simulink model "IndustrialMicrogrid"  (R2023a)
settings: Solver=FixedStepDiscrete  StartTime=0.0  StopTime=10  FixedStep=Ts  RelTol=1e-3
PostLoadFcn:
  | IndustrialMicrogridInputData
  | GfmGridFormingConverterInputParameters
model workspace (MAT data in the model file):
  caseNum = 2
undefined symbols (not defined in the file): base, BESS, DiscIntNeverNeededParam, grid, Grid, gridInverter, machine, microgrid, PV, PVInverter, PVTransformer, scrFactorRg, scrFactorXg, transformer, Ts
libraries: ee_lib x112, eeGeneralControl x104, nesl_utility_internal x64, simulink x56, nesl_utility x37, fl_lib x29, slpidlib x13, eeTransforms x11, eeTotalHarmonicDistorsion x8, eeRmsMeasurement x4, eeSinusoidalMeasurement x4, simulink_extras x2
(part 2 of 14)

== system IndustrialMicrogrid/MG2 PV Plant ==
  (500KWp PV) : Subsystem
      settings: PortSchema="{\"entries\":[{\"content\":{\"sides\":[{\"content\":{\"connectorIds\":[\"Out1\",\"In1\",\"LConn1\"]},\"type\":\"ConnectorPlacement.EquallySpacedRectSide\",\"uuid\":\"7b0e71bf-88d0-4fd9-b424-51733315768d\"},{\"content\":{\"side\":\"RIGHT\"},\"type\":\"ConnectorPlacement.EquallySpacedRectSide\",\"uuid\":\"454a206f-9a61-4ac7-86a8-f6508f61436e\"},{\"content\":{\"side\":\"TOP\"},\"type\":\"ConnectorPlacement.EquallySpacedRectSide\",\"uuid\":\"cf982e1c-b164-4d0a-abcb-f158cc5498a1\"}]},\"type\":\"ConnectorPlacement.EquallySpacedConnector\",\"uuid\":\"7d6089e9-e0b0-4b95-be20-3597ac4fefae\"}],\"packageUris\":[\"http://schema.mathworks.com/mf0/Connector/R2020b\"],\"version\":\"1.0\"}"
  4.16 kV/ 13.8 kV2 : ee_lib/Passive/Transformers/Two-Winding Transformer (Three-Phase)  SRated=PVTransformer.VA A*V  FRated=grid.frequency Hz  Winding1Connection=ee.enum.windingconnection.delta1  VRated1=PVTransformer.hv V  Winding2Connection=ee.enum.windingconnection.Yn  VRated2=PVTransformer.lv V  CoreType=ee.enum.coretype.threelimb  pu_Rw1=PVTransformer.windingResistance*1/2  pu_Rw2=PVTransformer.windingResistance*1/2  leakage_reactance_option=ee.enum.transformer_leakage.include  pu_Xl1=PVTransformer.windingLekageReactance*1/2  pu_Xl2=PVTransformer.windingLekageReactance*1/2  magnetizing_resistance_option=ee.enum.transformer_magnetizingResistance.exclude  pu_Rm=500  magnetizing_reactance_option=ee.enum.transformer_magnetizingReactance.exclude  saturation_option=ee.enum.transformer_saturation.exclude  pu_Xm=500  current_data=[0, .002, 1, 2]  magnetic_flux_data=[0, 1.2, 1.5, 1.51]  pu_X0=PVTransformer.zeroSequenceReactance*1.5  i1_specify=off  i1_priority=None  i1=[0, 0, 0] A  i1_nominal_specify=off  i1_nominal_unit=A  i1_nominal_value=1  i2_specify=off  i2_priority=None  i2=[0, 0, 0] A  i2_nominal_specify=off  i2_nominal_unit=A  i2_nominal_value=1  phi_specify=off  phi_priority=None  phi=[0, 0, 0]  phi_nominal_specify=off  phi_nominal_unit=1  phi_nominal_value=1  power_dissipated_specify=off  power_dissipated_priority=None  power_dissipated=0 W  power_dissipated_nominal_specify=off  power_dissipated_nominal_unit=W  power_dissipated_nominal_value=1
      settings: InternalSimscapePortConfiguration="{\"Bottom\":[],\"Left\":[{\"id\":\"N1\",\"label\":\"~1\",\"type\":\"foundation.electrical.three_phase\"}],\"Right\":[{\"id\":\"N2\",\"label\":\"~2\",\"type\":\"foundation.electrical.three_phase\"},{\"id\":\"n2\",\"label\":\"n2\",\"type\":\"foundation.electrical.electrical\"}],\"Top\":[]}"
  Bus Creator : BusCreator  Inputs=2
  Bus Selector : BusSelector  OutputSignals=Vmag
  CB4 : Subsystem
  Current and Voltage Sensor (Three-Phase)1 : ee_lib/Sensors & Transducers/Current and Voltage Sensor (Three-Phase)  vMeasurementType=ee.enum.vmeasurement.lg  outputUnit=ee.enum.unit.pu  SRated=PV.MVABaseNew A*V  VRated=PV.kVBaseNew V  I_specify=off  I_priority=None  I=[0, 0, 0] A  I_nominal_specify=off  I_nominal_unit=A  I_nominal_value=1  V_specify=off  V_priority=None  V=[0, 0, 0] V  V_nominal_specify=off  V_nominal_unit=V  V_nominal_value=1
      settings: InternalSimscapePortConfiguration="{\"Bottom\":[],\"Left\":[{\"id\":\"N1\",\"label\":\"~1\",\"type\":\"foundation.electrical.three_phase\"}],\"Right\":[{\"id\":\"V_output\",\"label\":\"V\",\"type\":\"output\"},{\"id\":\"I_output\",\"label\":\"I\",\"type\":\"output\"},{\"id\":\"N2\",\"label\":\"~2\",\"type\":\"foundation.electrical.three_phase\"}],\"Top\":[]}"
  Electrical Reference8 : fl_lib/Electrical/Electrical Elements/Electrical Reference
  PLL & Measurements2 : Subsystem
      settings: PortSchema="{\"entries\":[{\"content\":{\"sides\":[{\"content\":{\"connectorIds\":[\"Out1\",\"In1\"]},\"type\":\"ConnectorPlacement.EquallySpacedRectSide\",\"uuid\":\"76485780-20fe-4fcf-8224-69648da6ed2a\"},{\"content\":{\"connectorIds\":[],\"side\":\"RIGHT\"},\"type\":\"ConnectorPlacement.EquallySpacedRectSide\",\"uuid\":\"f19a6390-e634-42c7-8d46-4cd80cbab182\"},{\"content\":{\"connectorIds\":[],\"side\":\"TOP\"},\"type\":\"ConnectorPlacement.EquallySpacedRectSide\",\"uuid\":\"87682f72-1844-428e-be70-ad7ca3191ee3\"}]},\"type\":\"ConnectorPlacement.EquallySpacedConnector\",\"uuid\":\"f2136b07-48ec-402b-adb3-18c0bac2157c\"}],\"packageUris\":[\"http://schema.mathworks.com/mf0/Connector/R2020b\"],\"version\":\"1.0\"}"
  PS-Simulink Converter1 : nesl_utility/PS-Simulink Converter  PhysicalDomain=network_engine_domain  SubClassName=ps_output  LeftPortType=input  RightPortType=output  PseudoPeriodic=off  Frequencies=[]  VectorFormat=inherit  Unit=inherit  AffineConversion=off
  PS-Simulink Converter2 : nesl_utility/PS-Simulink Converter  PhysicalDomain=network_engine_domain  SubClassName=ps_output  LeftPortType=input  RightPortType=output  PseudoPeriodic=off  Frequencies=[]  VectorFormat=inherit  Unit=inherit  AffineConversion=off
  Step : Step  Time=microgrid.controller2PVBrk  Before=1  After=0  SampleTime=Ts
  Terminator : Terminator
  ~ : PMIOPort  Side=Left
  mPV : Outport
  wires:
  (500KWp PV)/1(mPV) -> Bus Creator/1  "mPV"
  PS-Simulink Converter1/1 -> Terminator/1
  Bus Creator/1 -> mPV/1
  Bus Selector/1 -> Bus Creator/2  "<Vmag>"
  Step/1 -> CB4/1(Input)
  PLL & Measurements2/1(Vbus) -> (500KWp PV)/1(Vbus), Bus Selector/1
  PS-Simulink Converter2/1 -> PLL & Measurements2/1(V)
  connections:
  Current and Voltage Sensor (Three-Phase)1/RConn3 -- 4.16 kV/ 13.8 kV2/RConn1
  Current and Voltage Sensor (Three-Phase)1/RConn2 -- PS-Simulink Converter1/LConn1
  CB4/LConn1 -- (500KWp PV)/LConn1
  4.16 kV/ 13.8 kV2/RConn2 -- Electrical Reference8/LConn1
  Current and Voltage Sensor (Three-Phase)1/RConn1 -- PS-Simulink Converter2/LConn1
  Current and Voltage Sensor (Three-Phase)1/LConn1 -- CB4/RConn1
  4.16 kV/ 13.8 kV2/LConn1 -- ~/RConn1

== system IndustrialMicrogrid/MG2 Power Center ==
  Bus Element In3 : Inport  PortName=ControlRoom  Element=PowerCenterBrk1
  Bus Element In1 : Inport  PortName=ControlRoom  Element=PowerCenterBrk2
  Bus Element In2 : Inport  PortName=ControlRoom  Element=PowerCenterDieselBrk
  Bus Element In4 : Inport  PortName=ControlRoom  Element=PowerCenterBrk3
  Circuit Breaker (Three-Phase){,1..3} (4 alike) : ee_lib/Switches & Breakers/Circuit Breaker (Three-Phase)  R_closed=0.001 Ohm  G_open=1e-6 1/Ohm  threshold=0.5 V  breaker_behavior=ee.enum.switches.breakerBehavior.zeroCrossingEnable
      settings: InternalSimscapePortConfiguration="{\"Bottom\":[],\"Left\":[{\"id\":\"vT\",\"label\":\"vT\",\"type\":\"input\"},{\"id\":\"N1\",\"label\":\"~1\",\"type\":\"foundation.electrical.three_phase\"}],\"Right\":[{\"id\":\"N2\",\"label\":\"~2\",\"type\":\"foundation.electrical.three_phase\"}],\"Top\":[]}"
  Diesel Generator : Subsystem
      mask Display: image('$imagefile'); % Use "Edit Image" on toolstrip to change.
  Diesel Measurements : Subsystem
  Fault (Three-Phase) : ee_lib/Utilities/Fault (Three-Phase)  fault_type_option=11  R_pn_fault=1e-3 Ohm  R_ng_fault=1e-3 Ohm  exposemeasurement=ee.enum.exposemeasurement.hidden  enable_external_fault=ee.enum.external_fault.hidden  fault_threshold=0.5  fault_condition=1  fault_resettable=0  enable_temporal_fault=1  fault_start_time=microgrid.controller2PowerCenterFault s  fault_duration=0.1 s  G_parasitic=1e-6 1/Ohm
      settings: InternalSimscapePortConfiguration="{\"Bottom\":[],\"Left\":[{\"id\":\"N\",\"label\":\"~\",\"type\":\"foundation.electrical.three_phase\"}],\"Right\":[],\"Top\":[]}"
  Line X/R=1.44 1 : ee_lib/Passive/RLC Assemblies/RLC (Three-Phase)  component_structure=ee.enum.rlc.structure.SeriesRL  R=microgrid.rLine*0.2 Ohm  L=microgrid.lLine*0.2 H  C=1 F  R_parasitic=1e-6 Ohm  G_parasitic=1e-5 1/Ohm  IL_specify=on  IL_priority=High  IL=[0, 0, 0] A  IL_nominal_specify=off  IL_nominal_unit=A  IL_nominal_value=1  VC_specify=on  VC_priority=High  VC=[0, 0, 0] V  VC_nominal_specify=off  VC_nominal_unit=V  VC_nominal_value=1
      settings: InternalSimscapePortConfiguration="{\"Bottom\":[],\"Left\":[{\"id\":\"N1\",\"label\":\"~1\",\"type\":\"foundation.electrical.three_phase\"}],\"Right\":[{\"id\":\"N2\",\"label\":\"~2\",\"type\":\"foundation.electrical.three_phase\"}],\"Top\":[]}"
  Line X/R=1.44 2 : ee_lib/Passive/RLC Assemblies/RLC (Three-Phase)  component_structure=ee.enum.rlc.structure.SeriesRL  R=microgrid.rLine*0.3 Ohm  L=microgrid.lLine*0.3 H  C=1 F  R_parasitic=1e-6 Ohm  G_parasitic=1e-5 1/Ohm  IL_specify=on  IL_priority=High  IL=[0, 0, 0] A  IL_nominal_specify=off  IL_nominal_unit=A  IL_nominal_value=1  VC_specify=on  VC_priority=High  VC=[0, 0, 0] V  VC_nominal_specify=off  VC_nominal_unit=V  VC_nominal_value=1
      settings: InternalSimscapePortConfiguration="{\"Bottom\":[],\"Left\":[{\"id\":\"N1\",\"label\":\"~1\",\"type\":\"foundation.electrical.three_phase\"}],\"Right\":[{\"id\":\"N2\",\"label\":\"~2\",\"type\":\"foundation.electrical.three_phase\"}],\"Top\":[]}"
  Line X/R=1.44 3 : ee_lib/Passive/RLC Assemblies/RLC (Three-Phase)  component_structure=ee.enum.rlc.structure.SeriesRL  R=microgrid.rLine*0.2 Ohm  L=microgrid.lLine*0.2 H  C=1 F  R_parasitic=1e-6 Ohm  G_parasitic=1e-5 1/Ohm  IL_specify=on  IL_priority=High  IL=[0, 0, 0] A  IL_nominal_specify=off  IL_nominal_unit=A  IL_nominal_value=1  VC_specify=on  VC_priority=High  VC=[0, 0, 0] V  VC_nominal_specify=off  VC_nominal_unit=V  VC_nominal_value=1
      settings: InternalSimscapePortConfiguration="{\"Bottom\":[],\"Left\":[{\"id\":\"N1\",\"label\":\"~1\",\"type\":\"foundation.electrical.three_phase\"}],\"Right\":[{\"id\":\"N2\",\"label\":\"~2\",\"type\":\"foundation.electrical.three_phase\"}],\"Top\":[]}"
  Low-Pass Filter (Discrete or Continuous) : eeGeneralControl/Low-Pass Filter (Discrete or Continuous)  K=1  T=0.1  B=inf  A=-inf  init_option=Inherited from block input  x0=0  Ts=Ts
  Low-Pass Filter (Discrete or Continuous)1 : eeGeneralControl/Low-Pass Filter (Discrete or Continuous)  K=1  T=0.1  B=inf  A=-inf  init_option=Inherited from block input  x0=0  Ts=Ts
  PS-Simulink Converter8 : nesl_utility_internal/PS-Simulink Converter  PhysicalDomain=network_engine_domain  SubClassName=ps_output  LeftPortType=input  RightPortType=output  PseudoPeriodic=off  Frequencies=[]  VectorFormat=1-D array  Unit=MW  AffineConversion=off
  PS-Simulink Converter9 : nesl_utility_internal/PS-Simulink Converter  PhysicalDomain=network_engine_domain  SubClassName=ps_output  LeftPortType=input  RightPortType=output  PseudoPeriodic=off  Frequencies=[]  VectorFormat=1-D array  Unit=MV*A  AffineConversion=off
  Power Sensor (Three-Phase)2 : ee_lib/Sensors & Transducers/Power Sensor (Three-Phase)  load_type=ee.enum.passive.type_balanced.balanced  f0=60 Hz  config=ee.enum.with_neutral.no  rho=1
      settings: InternalSimscapePortConfiguration="{\"Bottom\":[],\"Left\":[{\"id\":\"N1\",\"label\":\"~1\",\"type\":\"foundation.electrical.three_phase\"}],\"Right\":[{\"id\":\"N2\",\"label\":\"~2\",\"type\":\"foundation.electrical.three_phase\"}],\"Top\":[{\"id\":\"Pm\",\"label\":\"P\",\"type\":\"output\"},{\"id\":\"Qm\",\"label\":\"Q\",\"type\":\"output\"}]}"
  Simulink-PS Converter{,1..3} (4 alike) : nesl_utility_internal/Simulink-PS Converter  PhysicalDomain=network_engine_domain  SubClassName=ps_input  LeftPortType=input  RightPortType=output  PseudoPeriodic=off  Frequencies=[]  NoiseDistribution=none  NoiseParameters=[]  Unit=1  AffineConversion=off  FilteringAndDerivatives=provide  SimscapeFilterOrder=1  InputFilterTimeConstant=0.001  UdotUserProvided=0
  Transformer and Disconnectors : Subsystem
      mask Display: image('$imagefile'); % Use "Edit Image" on toolstrip to change.
  Two-Winding Transformer (Three-Phase)1 : ee_lib/Passive/Transformers/Two-Winding Transformer (Three-Phase)  SRated=microgrid.powerCenterTransformerRating A*V  FRated=microgrid.frequency Hz  Winding1Connection=ee.enum.windingconnection.Y  VRated1=microgrid.powerCenterTransformerPrimaryVoltage V  Winding2Connection=ee.enum.windingconnection.Y  VRated2=microgrid.powerCenterTransformerSecondaryVoltage V  CoreType=ee.enum.coretype.threelimb  pu_Rw1=microgrid.powerCenterPrimaryresistance  pu_Rw2=microgrid.powerCenterPrimaryreactance  leakage_reactance_option=ee.enum.transformer_leakage.include  pu_Xl1=microgrid.powerCenterSecondaryresistance  pu_Xl2=microgrid.powerCenterSecondaryreactance  magnetizing_resistance_option=ee.enum.transformer_magnetizingResistance.include  pu_Rm=500  magnetizing_reactance_option=ee.enum.transformer_magnetizingReactance.include  saturation_option=ee.enum.transformer_saturation.exclude  pu_Xm=500  current_data=[0, .002, 1, 2]  magnetic_flux_data=[0, 1.2, 1.5, 1.51]  pu_X0=0.5  i1_specify=on  i1_priority=None  i1=[0, 0, 0] A  i1_nominal_specify=off  i1_nominal_unit=A  i1_nominal_value=1  i2_specify=on  i2_priority=None  i2=[0, 0, 0] A  i2_nominal_specify=off  i2_nominal_unit=A  i2_nominal_value=1  phi_specify=off  phi_priority=None  phi=[0, 0, 0]  phi_nominal_specify=off  phi_nominal_unit=1  phi_nominal_value=1  power_dissipated_specify=off  power_dissipated_priority=None  power_dissipated=0 W  power_dissipated_nominal_specify=off  power_dissipated_nominal_unit=W  power_dissipated_nominal_value=1
      settings: InternalSimscapePortConfiguration="{\"Bottom\":[],\"Left\":[{\"id\":\"N1\",\"label\":\"~1\",\"type\":\"foundation.electrical.three_phase\"}],\"Right\":[{\"id\":\"N2\",\"label\":\"~2\",\"type\":\"foundation.electrical.three_phase\"}],\"Top\":[]}"
  Conn2 : PMIOPort  Side=Left
  ~ a : PMIOPort  Port=2  Side=Left
  " ~ " : PMIOPort  Port=3  Side=Right
  mdiesel : Outport
  Out Bus Element2 : Outport  Port=2  PortName=mtieline  Element=activepower
  Out Bus Element3 : Outport  Port=2  PortName=mtieline  Element=reactivepower
  wires:
  Bus Element In1/1 -> Simulink-PS Converter1/1
  Bus Element In3/1 -> Simulink-PS Converter/1
  Bus Element In2/1 -> Simulink-PS Converter2/1
  Diesel Measurements/1(mdiesel) -> mdiesel/1  "mDiesel"
  Bus Element In4/1 -> Simulink-PS Converter3/1
  PS-Simulink Converter8/1 -> Low-Pass Filter (Discrete or Continuous)/1
  Low-Pass Filter (Discrete or Continuous)1/1 -> Out Bus Element3/1
  PS-Simulink Converter9/1 -> Low-Pass Filter (Discrete or Continuous)1/1
  Low-Pass Filter (Discrete or Continuous)/1 -> Out Bus Element2/1
  connections:
  Line X/R=1.44 1/RConn1 -- Fault (Three-Phase)/LConn1 -- ~ a/RConn1
  Line X/R=1.44 3/RConn1 -- " ~ "/RConn1
  Circuit Breaker (Three-Phase)1/RConn1 -- Two-Winding Transformer (Three-Phase)1/LConn1
  Simulink-PS Converter/RConn1 -- Circuit Breaker (Three-Phase)/LConn1
  Circuit Breaker (Three-Phase)1/LConn2 -- Circuit Breaker (Three-Phase)3/LConn2 -- Circuit Breaker (Three-Phase)/RConn1
  Simulink-PS Converter1/RConn1 -- Circuit Breaker (Three-Phase)1/LConn1
  Line X/R=1.44 2/LConn1 -- Conn2/RConn1
  Diesel Generator/RConn1 -- Transformer and Disconnectors/LConn1
  Simulink-PS Converter2/RConn1 -- Circuit Breaker (Three-Phase)2/LConn1
  Circuit Breaker (Three-Phase)2/RConn1 -- Two-Winding Transformer (Three-Phase)1/RConn1 -- Line X/R=1.44 3/LConn1
  Transformer and Disconnectors/RConn1 -- Diesel Measurements/LConn1
  Diesel Measurements/RConn1 -- Circuit Breaker (Three-Phase)2/LConn2
  Circuit Breaker (Three-Phase)3/RConn1 -- Line X/R=1.44 1/LConn1
  Simulink-PS Converter3/RConn1 -- Circuit Breaker (Three-Phase)3/LConn1
  PS-Simulink Converter9/LConn1 -- Power Sensor (Three-Phase)2/LConn3
  PS-Simulink Converter8/LConn1 -- Power Sensor (Three-Phase)2/LConn2
  Power Sensor (Three-Phase)2/LConn1 -- Line X/R=1.44 2/RConn1
  Power Sensor (Three-Phase)2/RConn1 -- Circuit Breaker (Three-Phase)/LConn2

== system IndustrialMicrogrid/MG2 Primary Substation ==
  ControlRoom : Inport
  BESS and Controller 2 : Subsystem
  Bus Creator : BusCreator  Inputs=2
  Bus Selector : BusSelector  OutputSignals=Substation2Brk
  Circuit Breaker (Three-Phase) : ee_lib/Switches & Breakers/Circuit Breaker (Three-Phase)  R_closed=0.001 Ohm  G_open=1e-6 1/Ohm  threshold=0.5 V  breaker_behavior=ee.enum.switches.breakerBehavior.zeroCrossingEnable
      settings: InternalSimscapePortConfiguration="{\"Bottom\":[],\"Left\":[{\"id\":\"vT\",\"label\":\"vT\",\"type\":\"input\"},{\"id\":\"N1\",\"label\":\"~1\",\"type\":\"foundation.electrical.three_phase\"}],\"Right\":[{\"id\":\"N2\",\"label\":\"~2\",\"type\":\"foundation.electrical.three_phase\"}],\"Top\":[]}"
  Microgrid Controller 2 : Subsystem
  PCC Measurements and PCC Breaker : Subsystem
      mask Display: image('$imagefile'); % Use "Edit Image" on toolstrip to change.
  Simulink-PS Converter : nesl_utility_internal/Simulink-PS Converter  PhysicalDomain=network_engine_domain  SubClassName=ps_input  LeftPortType=input  RightPortType=output  PseudoPeriodic=off  Frequencies=[]  NoiseDistribution=none  NoiseParameters=[]  Unit=1  AffineConversion=off  FilteringAndDerivatives=provide  SimscapeFilterOrder=1  InputFilterTimeConstant=0.001  UdotUserProvided=0
  Transformer and Disconnectors : Subsystem
      mask Display: image('$imagefile'); % Use "Edit Image" on toolstrip to change.
  ~ : PMIOPort  Side=Left
  "~ " : PMIOPort  Port=2  Side=Right
  MGController2 : Outport
  wires:
  Bus Creator/1 -> MGController2/1
  BESS and Controller 2/1(mBESS) -> Bus Creator/1, [BESS2]  "BESS2"
  PCC Measurements and PCC Breaker/1(" mPCC2") -> Microgrid Controller 2/3("mPCC2 ")
  [CtrlRoom] -> Bus Selector/1
  Bus Selector/1 -> Simulink-PS Converter/1  "<Substation2Brk>"
  [CtrlRoom] -> BESS and Controller 2/1(CntrlRmIN)
  [BESS2] -> Microgrid Controller 2/2(BESS 2)
  Microgrid Controller 2/4(MGCtrl) -> [Controller]
  [Controller] -> Bus Creator/2
  ControlRoom/1 -> [CtrlRoom]
  [CtrlRoom] -> Microgrid Controller 2/1(CntrlRmIN)
  Microgrid Controller 2/5(BrkCtrl) -> [cBreaker]
  [cBreaker] -> PCC Measurements and PCC Breaker/1(cBreaker)
  Microgrid Controller 2/1(PQref) -> BESS and Controller 2/2(PQref)
  Microgrid Controller 2/2(Vref) -> BESS and Controller 2/3(Vref)
  Microgrid Controller 2/3(fref) -> BESS and Controller 2/4(f0)
  connections:
  ~/RConn1 -- Transformer and Disconnectors/LConn1
  Transformer and Disconnectors/RConn1 -- PCC Measurements and PCC Breaker/LConn1
  PCC Measurements and PCC Breaker/RConn1 -- Circuit Breaker (Three-Phase)/LConn2 -- BESS and Controller 2/LConn1
  Simulink-PS Converter/RConn1 -- Circuit Breaker (Three-Phase)/LConn1
  "~ "/RConn1 -- Circuit Breaker (Three-Phase)/RConn1

== system IndustrialMicrogrid/MG2 Processing, Lighting and Auxiliary Loads ==
  Bus Element In1 : Inport  PortName=ControlRoom  Element=Load3Control
  Bus Element In4 : Inport  PortName=ControlRoom  Element=Load5Control
  Bus Element In3 : Inport  PortName=ControlRoom  Element=Load4aControl
  Bus Element In2 : Inport  PortName=ControlRoom  Element=Load4bControl
  Circuit Breaker (Three-Phase){1..4} (4 alike) : ee_lib/Switches & Breakers/Circuit Breaker (Three-Phase)  R_closed=0.001 Ohm  G_open=1e-6 1/Ohm  threshold=0.5 V  breaker_behavior=ee.enum.switches.breakerBehavior.zeroCrossingEnable
      settings: InternalSimscapePortConfiguration="{\"Bottom\":[],\"Left\":[{\"id\":\"vT\",\"label\":\"vT\",\"type\":\"input\"},{\"id\":\"N1\",\"label\":\"~1\",\"type\":\"foundation.electrical.three_phase\"}],\"Right\":[{\"id\":\"N2\",\"label\":\"~2\",\"type\":\"foundation.electrical.three_phase\"}],\"Top\":[]}"
  Electrical Reference1 : fl_lib/Electrical/Electrical Elements/Electrical Reference
  Electrical Reference2 : fl_lib/Electrical/Electrical Elements/Electrical Reference
  Electrical Reference5 : fl_lib/Electrical/Electrical Elements/Electrical Reference
  Load Measurements1 : Subsystem
      settings: PortSchema="{\"entries\":[{\"content\":{\"sides\":[{\"content\":{\"connectorIds\":[\"LConn1\"]},\"type\":\"ConnectorPlacement.EquallySpacedRectSide\",\"uuid\":\"d870a913-f96e-493f-ac0f-f00d694ce040\"},{\"content\":{\"connectorIds\":[\"Out1\"],\"side\":\"RIGHT\"},\"type\":\"ConnectorPlacement.EquallySpacedRectSide\",\"uuid\":\"12eea89c-1ef8-4155-8c58-3c970c5d9b18\"},{\"content\":{\"connectorIds\":[],\"side\":\"TOP\"},\"type\":\"ConnectorPlacement.EquallySpacedRectSide\",\"uuid\":\"8c8b4bd0-9ee8-4a98-bcb2-09acde5bae56\"},{\"content\":{\"connectorIds\":[\"RConn1\"],\"side\":\"BOTTOM\"},\"type\":\"ConnectorPlacement.EquallySpacedRectSide\",\"uuid\":\"443bcb6e-ffa1-4f95-8c19-122149ac17cf\"}]},\"type\":\"ConnectorPlacement.EquallySpacedConnector\",\"uuid\":\"4cf8469f-5e58-4383-9537-851b6a4abf90\"}],\"packageUris\":[\"http://schema.mathworks.com/mf0/Connector/R2020b\"],\"version\":\"1.0\"}"
  Load for auxiliary : ee_lib/Passive/RLC Assemblies/Wye-Connected Load  parameterization=ee.enum.rlc.parameterization.ratedpower  component_structure=ee.enum.rlc.structure.C  component_structure_PQ=ee.enum.rlc.structure.SeriesRL  R=1 Ohm  L=0.001 H  C=1e-6 F  VRated=microgrid.powerCenterVoltage V  FRated=microgrid.frequency Hz  P=microgrid.pLoad22 W  Qpos=microgrid.qLoad22 A*V  Qneg=-3000 A*V  R_parasitic=1e-6 Ohm  G_parasitic=1e-6 1/Ohm  R_parasitic_PQ=1e-6 Ohm  G_parasitic_PQ=1e-6 1/Ohm  Vmag0=0 V  Vang0=0 deg  Freq0=microgrid.frequency Hz  IL_specify=on  IL_priority=High  IL=[ 0 0 0 ] A  IL_nominal_specify=off  IL_nominal_unit=A  IL_nominal_value=1  VC_specify=on  VC_priority=High  VC=[ 0 0 0 ] V  VC_nominal_specify=off  VC_nominal_unit=V  VC_nominal_value=1
  Load for auxiliary1 : ee_lib/Passive/RLC Assemblies/Wye-Connected Load  parameterization=ee.enum.rlc.parameterization.ratedpower  component_structure=ee.enum.rlc.structure.C  component_structure_PQ=ee.enum.rlc.structure.SeriesRL  R=1 Ohm  L=0.001 H  C=1e-6 F  VRated=microgrid.powerCenterVoltage V  FRated=microgrid.frequency Hz  P=microgrid.pLoad33 W  Qpos=microgrid.qLoad33 A*V  Qneg=-3000 A*V  R_parasitic=1e-6 Ohm  G_parasitic=1e-6 1/Ohm  R_parasitic_PQ=1e-6 Ohm  G_parasitic_PQ=1e-6 1/Ohm  Vmag0=0 V  Vang0=0 deg  Freq0=microgrid.frequency Hz  IL_specify=on  IL_priority=High  IL=[ 0 0 0 ] A  IL_nominal_specify=off  IL_nominal_unit=A  IL_nominal_value=1  VC_specify=on  VC_priority=High  VC=[ 0 0 0 ] V  VC_nominal_specify=off  VC_nominal_unit=V  VC_nominal_value=1
  Load for lights : ee_lib/Passive/RLC Assemblies/Wye-Connected Load  parameterization=ee.enum.rlc.parameterization.ratedpower  component_structure=ee.enum.rlc.structure.C  component_structure_PQ=ee.enum.rlc.structure.SeriesRL  R=1 Ohm  L=0.001 H  C=1e-6 F  VRated=microgrid.powerCenterVoltage V  FRated=microgrid.frequency Hz  P=microgrid.pLoad21 W  Qpos=microgrid.qLoad21 A*V  Qneg=-3000 A*V  R_parasitic=1e-6 Ohm  G_parasitic=1e-6 1/Ohm  R_parasitic_PQ=1e-6 Ohm  G_parasitic_PQ=1e-6 1/Ohm  Vmag0=0 V  Vang0=0 deg  Freq0=microgrid.frequency Hz  IL_specify=on  IL_priority=High  IL=[ 0 0 0 ] A  IL_nominal_specify=off  IL_nominal_unit=A  IL_nominal_value=1  VC_specify=on  VC_priority=High  VC=[ 0 0 0 ] V  VC_nominal_specify=off  VC_nominal_unit=V  VC_nominal_value=1
  Motor Loads : Subsystem
  RLC (Three-Phase) : ee_lib/Passive/RLC Assemblies/RLC (Three-Phase)  component_structure=ee.enum.rlc.structure.SeriesRL  R=1 Ohm  L=5e-3 H  C=1e-6 F  R_parasitic=0 Ohm  G_parasitic=0 1/Ohm  IL_specify=off  IL_priority=High  IL=[0, 0, 0] A  IL_nominal_specify=off  IL_nominal_unit=A  IL_nominal_value=1  VC_specify=off  VC_priority=High  VC=[0, 0, 0] V  VC_nominal_specify=off  VC_nominal_unit=V  VC_nominal_value=1
      settings: InternalSimscapePortConfiguration="{\"Bottom\":[],\"Left\":[{\"id\":\"N1\",\"label\":\"~1\",\"type\":\"foundation.electrical.three_phase\"}],\"Right\":[{\"id\":\"N2\",\"label\":\"~2\",\"type\":\"foundation.electrical.three_phase\"}],\"Top\":[]}"
  Simulink-PS Converter{1..4} (4 alike) : nesl_utility_internal/Simulink-PS Converter  PhysicalDomain=network_engine_domain  SubClassName=ps_input  LeftPortType=input  RightPortType=output  PseudoPeriodic=off  Frequencies=[]  NoiseDistribution=none  NoiseParameters=[]  Unit=1  AffineConversion=off  FilteringAndDerivatives=provide  SimscapeFilterOrder=1  InputFilterTimeConstant=0.001  UdotUserProvided=0
  ~ : PMIOPort  Side=Left
  mLoad2 : Outport
  wires:
  Load Measurements1/1(mLoad2) -> mLoad2/1
  Bus Element In1/1 -> Simulink-PS Converter3/1
  Bus Element In3/1 -> Simulink-PS Converter1/1
  Bus Element In4/1 -> Simulink-PS Converter2/1
  Bus Element In2/1 -> Simulink-PS Converter4/1
  connections:
  Electrical Reference2/LConn1 -- Load for lights/RConn1
  Simulink-PS Converter3/RConn1 -- Circuit Breaker (Three-Phase)1/LConn1
  Simulink-PS Converter1/RConn1 -- Circuit Breaker (Three-Phase)2/LConn1
  ~/RConn1 -- Load Measurements1/LConn1
  Circuit Breaker (Three-Phase)1/RConn1 -- Load for lights/LConn1
  Load for auxiliary/LConn1 -- Circuit Breaker (Three-Phase)2/RConn1
  Load for auxiliary/RConn1 -- Electrical Reference5/LConn1
  RLC (Three-Phase)/RConn1 -- Circuit Breaker (Three-Phase)3/LConn2
  Simulink-PS Converter2/RConn1 -- Circuit Breaker (Three-Phase)3/LConn1
  Load Measurements1/RConn1 -- Circuit Breaker (Three-Phase)2/LConn2 -- Circuit Breaker (Three-Phase)4/LConn2 -- RLC (Three-Phase)/LConn1 -- Circuit Breaker (Three-Phase)1/LConn2
  Load for auxiliary1/RConn1 -- Electrical Reference1/LConn1
  Load for auxiliary1/LConn1 -- Circuit Breaker (Three-Phase)4/RConn1
  Simulink-PS Converter4/RConn1 -- Circuit Breaker (Three-Phase)4/LConn1
  Motor Loads/RConn1 -- Circuit Breaker (Three-Phase)3/RConn1

== system IndustrialMicrogrid/Operator Room ==
  mLoad : Inport
  MGController1 : Inport  Port=2
  mTieline1 : Inport  Port=3
  MGController2 : Inport  Port=4
  mPV : Inport  Port=5
  mPowerCenter : Inport  Port=6
  mLoad2 : Inport  Port=7
  mLoad3 : Inport  Port=8
  Bus Creator : BusCreator  Inputs=9
  Bus Creator1 : BusCreator  Inputs=7
  Bus Selector7 : BusSelector  OutputSignals=mDiesel,mTieline
  OperatorControlRoom : Subsystem
      settings: PortSchema="{\"entries\":[{\"content\":{\"sides\":[{\"content\":{\"connectorIds\":[\"Out1\",\"Out2\"]},\"type\":\"ConnectorPlacement.EquallySpacedRectSide\",\"uuid\":\"36e3c748-e70d-4376-8c54-bee35c2cf55e\"},{\"content\":{\"connectorIds\":[\"In1\",\"In2\",\"In3\",\"In4\",\"In5\",\"In6\",\"In7\",\"In8\",\"In9\"],\"side\":\"RIGHT\"},\"type\":\"ConnectorPlacement.EquallySpacedRectSide\",\"uuid\":\"3af4b9ea-3351-4c6c-90c1-760bf6d2a862\"},{\"content\":{\"side\":\"TOP\"},\"type\":\"ConnectorPlacement.EquallySpacedRectSide\",\"uuid\":\"c84439f5-3dbb-4f33-afb8-95498296d6fa\"}]},\"type\":\"ConnectorPlacement.EquallySpacedConnector\",\"uuid\":\"cafa6b3a-2446-4c45-9268-4fc6f6c2350c\"}],\"packageUris\":[\"http://schema.mathworks.com/mf0/Connector/R2020b\"],\"version\":\"1.0\"}"
  Signal Selector : Subsystem
  OperatorRoom : Outport
  OperatorRoomResult : Outport  Port=2
  wires:
  Signal Selector/6("Processing, and Auxiliary Loads ") -> Bus Creator1/6  "Auxiliary Loads"
  MGController2/1 -> Bus Creator/3, OperatorControlRoom/3(MGController2)  "MGController2"
  OperatorControlRoom/1(Control Room MG1) -> Signal Selector/1(Control Room MG1)
  Signal Selector/5(Drilling Load) -> Bus Creator1/5  "Drilling Load"
  Signal Selector/4(Power Center) -> Bus Creator1/4  "Power Center"
  Bus Selector7/1 -> Bus Creator/8, OperatorControlRoom/8(mDiesel)  "<mDiesel>"
  Signal Selector/1(Primary Substation 1) -> Bus Creator1/1  "Primary Substation 1"
  MGController1/1 -> Bus Creator/5, OperatorControlRoom/5(MGController1)  "MGController1"
  mLoad2/1 -> Bus Creator/2, OperatorControlRoom/2(mLoad2)  "mLoad2"
  mLoad/1 -> Bus Creator/1, OperatorControlRoom/1(mLoad)  "mLoad"
  mPV/1 -> Bus Creator/4, OperatorControlRoom/4(mPV)  "mPV"
  Signal Selector/3(Unit Substation) -> Bus Creator1/3  "Unit Substation"
  Signal Selector/7(Portable Substation) -> Bus Creator1/7  "Portable Substation"
  Signal Selector/2(Primary Substation 2) -> Bus Creator1/2  "Primary Substation 2"
  OperatorControlRoom/2(Control Room MG2) -> Signal Selector/2(Control Room MG2)
  mLoad3/1 -> Bus Creator/7, OperatorControlRoom/7(mLoad3)  "mLoad3"
  mPowerCenter/1 -> Bus Selector7/1  "PowerCenter"
  Bus Selector7/2 -> Bus Creator/9, OperatorControlRoom/9(Tieline)  "<mTieline>"
  Bus Creator1/1 -> OperatorRoom/1
  mTieline1/1 -> Bus Creator/6, OperatorControlRoom/6(Tieline1)  "mTieline1"
  Bus Creator/1 -> OperatorRoomResult/1

== system IndustrialMicrogrid/Selected Results ==
  OperatorRoom : Inport
  Bus Selector1 : BusSelector  OutputSignals=MGController2,mLoad2,mPV,mDiesel
  Bus Selector7 : BusSelector  OutputSignals=MGController1,mLoad
  MG1 : Subsystem
  MG2 : Subsystem
  OperatorRoom1 : InportShadow
  wires:
  Bus Selector7/2 -> MG1/2(mLoad)  "<mLoad>"
  Bus Selector7/1 -> MG1/1(MGController1)  "<MGController1>"
  Bus Selector1/1 -> MG2/1(MGController2)  "<MGController2>"
  Bus Selector1/2 -> MG2/2(mLoad2)  "<mLoad2>"
  Bus Selector1/3 -> MG2/3(mPV)  "<mPV>"
  Bus Selector1/4 -> MG2/4(mdiesel)  "<mDiesel>"
  OperatorRoom/1 -> Bus Selector7/1
  OperatorRoom1/1 -> Bus Selector1/1

== system IndustrialMicrogrid/MG1 Drilling Loads/Load Measurements1 ==
  Current and Voltage Sensor (Three-Phase)2 : ee_lib/Sensors & Transducers/Current and Voltage Sensor (Three-Phase)  vMeasurementType=ee.enum.vmeasurement.ll  outputUnit=ee.enum.unit.pu  SRated=1e6 A*V  VRated=microgrid.unitSubstationVoltage V  I_specify=off  I_priority=None  I=[0, 0, 0] A  I_nominal_specify=off  I_nominal_unit=A  I_nominal_value=1  V_specify=off  V_priority=None  V=[0, 0, 0] V  V_nominal_specify=off  V_nominal_unit=V  V_nominal_value=1
      settings: InternalSimscapePortConfiguration="{\"Bottom\":[],\"Left\":[{\"id\":\"N1\",\"label\":\"~1\",\"type\":\"foundation.electrical.three_phase\"}],\"Right\":[{\"id\":\"V_output\",\"label\":\"V\",\"type\":\"output\"},{\"id\":\"I_output\",\"label\":\"I\",\"type\":\"output\"},{\"id\":\"N2\",\"label\":\"~2\",\"type\":\"foundation.electrical.three_phase\"}],\"Top\":[]}"
  Gain : Gain  Gain=sqrt(2)
  Gain1 : Gain  Gain=sqrt(2)
  Line Voltage Sensor (Three-Phase) : ee_lib/Sensors & Transducers/Line Voltage Sensor (Three-Phase)
  Low-Pass Filter (Discrete or Continuous)1 : eeGeneralControl/Low-Pass Filter (Discrete or Continuous)  K=1  T=0.02  B=inf  A=-inf  init_option=Inherited from block input  x0=0  Ts=Ts
  Low-Pass Filter (Discrete or Continuous)2 : eeGeneralControl/Low-Pass Filter (Discrete or Continuous)  K=1  T=0.02  B=inf  A=-inf  init_option=Inherited from block input  x0=0  Ts=Ts
  PS-Simulink Converter : nesl_utility/PS-Simulink Converter  PhysicalDomain=network_engine_domain  SubClassName=ps_output  LeftPortType=input  RightPortType=output  PseudoPeriodic=off  Frequencies=[]  VectorFormat=inherit  Unit=inherit  AffineConversion=off
  PS-Simulink Converter1 : nesl_utility_internal/PS-Simulink Converter  PhysicalDomain=network_engine_domain  SubClassName=ps_output  LeftPortType=input  RightPortType=output  PseudoPeriodic=off  Frequencies=[]  VectorFormat=1-D array  Unit=inherit  AffineConversion=off
  PS-Simulink Converter12 : nesl_utility_internal/PS-Simulink Converter  PhysicalDomain=network_engine_domain  SubClassName=ps_output  LeftPortType=input  RightPortType=output  PseudoPeriodic=off  Frequencies=[]  VectorFormat=1-D array  Unit=V  AffineConversion=off
  PS-Simulink Converter13 : nesl_utility_internal/PS-Simulink Converter  PhysicalDomain=network_engine_domain  SubClassName=ps_output  LeftPortType=input  RightPortType=output  PseudoPeriodic=off  Frequencies=[]  VectorFormat=1-D array  Unit=A  AffineConversion=off
  PS-Simulink Converter2 : nesl_utility_internal/PS-Simulink Converter  PhysicalDomain=network_engine_domain  SubClassName=ps_output  LeftPortType=input  RightPortType=output  PseudoPeriodic=off  Frequencies=[]  VectorFormat=1-D array  Unit=inherit  AffineConversion=off
  PS-Simulink Converter6 : nesl_utility_internal/PS-Simulink Converter  PhysicalDomain=network_engine_domain  SubClassName=ps_output  LeftPortType=input  RightPortType=output  PseudoPeriodic=off  Frequencies=[]  VectorFormat=1-D array  Unit=MW  AffineConversion=off
  PS-Simulink Converter7 : nesl_utility_internal/PS-Simulink Converter  PhysicalDomain=network_engine_domain  SubClassName=ps_output  LeftPortType=input  RightPortType=output  PseudoPeriodic=off  Frequencies=[]  VectorFormat=1-D array  Unit=MV*A  AffineConversion=off
  Power Sensor (Three-Phase)1 : ee_lib/Sensors & Transducers/Power Sensor (Three-Phase)  load_type=ee.enum.passive.type_balanced.balanced  f0=60 Hz  config=ee.enum.with_neutral.no  rho=1
      settings: InternalSimscapePortConfiguration="{\"Bottom\":[],\"Left\":[{\"id\":\"N1\",\"label\":\"~1\",\"type\":\"foundation.electrical.three_phase\"}],\"Right\":[{\"id\":\"N2\",\"label\":\"~2\",\"type\":\"foundation.electrical.three_phase\"}],\"Top\":[{\"id\":\"Pm\",\"label\":\"P\",\"type\":\"output\"},{\"id\":\"Qm\",\"label\":\"Q\",\"type\":\"output\"}]}"
  RMS Measurement : eeRmsMeasurement/RMS Measurement  LabelModeActiveChoice=Total  F=60  SpecifyHarmonics=off  K=[0 1 2]  Ts=Ts
      settings: LibrarySourceBlock=|
      | ee_sl_lib/Measurements/RMS
      | Measurement
  RMS Measurement1 : eeRmsMeasurement/RMS Measurement  LabelModeActiveChoice=Total  F=60  SpecifyHarmonics=off  K=[0 1 2]  Ts=Ts
      settings: LibrarySourceBlock=|
      | ee_sl_lib/Measurements/RMS
      | Measurement
  Scope : Scope
  a2 : PMIOPort  Side=Left
  Conn2 : PMIOPort  Port=2  Side=Right
  Out Bus Element : Outport  PortName=mLoad  Element=active power
  Out Bus Element1 : Outport  PortName=mLoad  Element=reactive power
  Out Bus Element2 : Outport  PortName=mLoad  Element=voltage
  Out Bus Element3 : Outport  PortName=mLoad  Element=current
  Out Bus Element4 : Outport  PortName=mLoad  Element=voltageRMS
  Out Bus Element5 : Outport  PortName=mLoad  Element=currentRMS
  wires:
  PS-Simulink Converter12/1 -> Out Bus Element2/1
  PS-Simulink Converter13/1 -> Out Bus Element3/1
  PS-Simulink Converter7/1 -> Low-Pass Filter (Discrete or Continuous)2/1
  PS-Simulink Converter6/1 -> Low-Pass Filter (Discrete or Continuous)1/1
  PS-Simulink Converter1/1 -> RMS Measurement/1
  PS-Simulink Converter2/1 -> RMS Measurement1/1
  Low-Pass Filter (Discrete or Continuous)1/1 -> Out Bus Element/1
  Low-Pass Filter (Discrete or Continuous)2/1 -> Out Bus Element1/1
  RMS Measurement/1 -> Gain/1
  RMS Measurement1/1 -> Gain1/1
  PS-Simulink Converter/1 -> Scope/1
  Gain/1 -> Out Bus Element4/1
  Gain1/1 -> Out Bus Element5/1
  connections:
  Power Sensor (Three-Phase)1/LConn3 -- PS-Simulink Converter7/LConn1
  Power Sensor (Three-Phase)1/LConn2 -- PS-Simulink Converter6/LConn1
  Current and Voltage Sensor (Three-Phase)2/RConn3 -- Conn2/RConn1
  a2/RConn1 -- Power Sensor (Three-Phase)1/LConn1 -- Line Voltage Sensor (Three-Phase)/LConn1
  Current and Voltage Sensor (Three-Phase)2/RConn1 -- PS-Simulink Converter12/LConn1 -- PS-Simulink Converter1/LConn1
  Current and Voltage Sensor (Three-Phase)2/RConn2 -- PS-Simulink Converter2/LConn1 -- PS-Simulink Converter13/LConn1
  Power Sensor (Three-Phase)1/RConn1 -- Current and Voltage Sensor (Three-Phase)2/LConn1
  PS-Simulink Converter/LConn1 -- Line Voltage Sensor (Three-Phase)/RConn1

== system IndustrialMicrogrid/MG1 Drilling Loads/Subsystem2 ==
  ASM measurement : ee_lib/Electromechanical/Asynchronous/Induction Machine Measurement  output_idx=11
      settings: InternalSimscapePortConfiguration="{\"Bottom\":[],\"Left\":[{\"id\":\"pu_input\",\"label\":\"pu\",\"type\":\"input\"}],\"Right\":[{\"id\":\"pu_output\",\"label\":\"o\",\"type\":\"output\"}],\"Top\":[]}"
  ASM measurement1 : ee_lib/Electromechanical/Asynchronous/Induction Machine Measurement  output_idx=12
      settings: InternalSimscapePortConfiguration="{\"Bottom\":[],\"Left\":[{\"id\":\"pu_input\",\"label\":\"pu\",\"type\":\"input\"}],\"Right\":[{\"id\":\"pu_output\",\"label\":\"o\",\"type\":\"output\"}],\"Top\":[]}"
  ASM measurement2 : ee_lib/Electromechanical/Asynchronous/Induction Machine Measurement  output_idx=12
      settings: InternalSimscapePortConfiguration="{\"Bottom\":[],\"Left\":[{\"id\":\"pu_input\",\"label\":\"pu\",\"type\":\"input\"}],\"Right\":[{\"id\":\"pu_output\",\"label\":\"o\",\"type\":\"output\"}],\"Top\":[]}"
  Asynchronous Machine Squirrel Cage (fundamental) : ee_lib/Electromechanical/Asynchronous/Induction Machine Squirrel Cage  port_option=ee.enum.threePhasePort.composite  SRated=132000 V*A  VRated=microgrid.unitSubstationVoltage V  FRated=grid.frequency Hz  nPolePairs=2  param_unit=ee.enum.unit.si  squirrel_cage=ee.enum.squirrelcage.Single  zero_sequence=ee.enum.park.zerosequence.exclude  initialization_option=ee.enum.asm.initialization.fluxvariables  Rs=0.016744 Ohm  Xls=0.035490 Ohm  pu_Rs=0.0258  pu_Lls=0.0413  Rrd=0.009857 Ohm  Xlrd=0.04280 Ohm  pu_Rrd=0.0145  pu_Llrd=0.0424  Rrd1=0.28 Ohm  Xlrd1=0.82 Ohm  Rrd2=0.28 Ohm  Xlrd2=0.82 Ohm  pu_Rrd1=0.0290  pu_Llrd1=0.0848  pu_Rrd2=0.0290  pu_Llrd2=0.0848  Xm=111.90 Ohm  pu_Lm=1.7562  X0=0.4 Ohm  pu_L0=0.0413  saturation_option=ee.enum.saturation.exclude  saturation_i=[0, 4, 9, 18, 25, 34, 50, 68, 95, 120] A  saturation_v=[0, 88, 154, 198, 220, 242, 264, 286, 308, 327] V  pu_saturation_i=[0, .176, .396, .792, 1.1, 1.496, 2.2, 2.992, 4.18, 5.28]  pu_saturation_v=[0, .4, .7, .9, 1, 1.1, 1.2, 1.3, 1.4, 1.4864]  connection_option=ee.enum.Connection.delta1  angular_position_specify=off  angular_position_priority=None  angular_position=0 deg  angular_position_nominal_specify=off  angular_position_nominal_unit=deg  angular_position_nominal_value=1  pu_psids_specify=off  pu_psids_priority=None  pu_psids=0  pu_psids_nominal_specify=off  pu_psids_nominal_unit=1  pu_psids_nominal_value=1  pu_psiqs_specify=off  pu_psiqs_priority=None  pu_psiqs=0  pu_psiqs_nominal_specify=off  pu_psiqs_nominal_unit=1  pu_psiqs_nominal_value=1  pu_psi0s_specify=off  pu_psi0s_priority=None  pu_psi0s=0  pu_psi0s_nominal_specify=off  pu_psi0s_nominal_unit=1  pu_psi0s_nominal_value=1  pu_psidr_specify=off  pu_psidr_priority=None  pu_psidr=0  pu_psidr_nominal_specify=off  pu_psidr_nominal_unit=1  pu_psidr_nominal_value=1  pu_psiqr_specify=off  pu_psiqr_priority=None  pu_psiqr=0  pu_psiqr_nominal_specify=off  pu_psiqr_nominal_unit=1  pu_psiqr_nominal_value=1  pu_psidr1_specify=off  pu_psidr1_priority=None  pu_psidr1=0  pu_psidr1_nominal_specify=off  pu_psidr1_nominal_unit=1  pu_psidr1_nominal_value=1  pu_psiqr1_specify=off  pu_psiqr1_priority=None  pu_psiqr1=0  pu_psiqr1_nominal_specify=off  pu_psiqr1_nominal_unit=1  pu_psiqr1_nominal_value=1  pu_psidr2_specify=off  pu_psidr2_priority=None  pu_psidr2=0  pu_psidr2_nominal_specify=off  pu_psidr2_nominal_unit=1  pu_psidr2_nominal_value=1  pu_psiqr2_specify=off  pu_psiqr2_priority=None  pu_psiqr2=0  pu_psiqr2_nominal_specify=off  pu_psiqr2_nominal_unit=1  pu_psiqr2_nominal_value=1  psids_specify=off  psids_priority=None  psids=0 Wb  psids_nominal_specify=off  psids_nominal_unit=Wb  psids_nominal_value=1  psiqs_specify=off  psiqs_priority=None  psiqs=0 Wb  psiqs_nominal_specify=off  psiqs_nominal_unit=Wb  psiqs_nominal_value=1  psi0s_specify=off  psi0s_priority=None  psi0s=0 Wb  psi0s_nominal_specify=off  psi0s_nominal_unit=Wb  psi0s_nominal_value=1  psidr_specify=off  psidr_priority=None  psidr=0 Wb  psidr_nominal_specify=off  psidr_nominal_unit=Wb  psidr_nominal_value=1  psiqr_specify=off  psiqr_priority=None  psiqr=0 Wb  psiqr_nominal_specify=off  psiqr_nominal_unit=Wb  psiqr_nominal_value=1  psidr1_specify=off  psidr1_priority=None  psidr1=0 Wb  psidr1_nominal_specify=off  psidr1_nominal_unit=Wb  psidr1_nominal_value=1  psiqr1_specify=off  psiqr1_priority=None  psiqr1=0 Wb  psiqr1_nominal_specify=off  psiqr1_nominal_unit=Wb  psiqr1_nominal_value=1  psidr2_specify=off  psidr2_priority=None  psidr2=0 Wb  psidr2_nominal_specify=off  psidr2_nominal_unit=Wb  psidr2_nominal_value=1  psiqr2_specify=off  psiqr2_priority=None  psiqr2=0 Wb  psiqr2_nominal_specify=off  psiqr2_nominal_unit=Wb  psiqr2_nominal_value=1  slip_specify=off  slip_priority=None  slip=0  slip_nominal_specify=off  slip_nominal_unit=1  slip_nominal_value=1  real_power_generated_specify=off  real_power_generated_priority=None  real_power_generated=0 W  real_power_generated_nominal_specify=off  real_power_generated_nominal_unit=W  real_power_generated_nominal_value=1  mechanical_power_consumed_specify=off  mechanical_power_consumed_priority=None  mechanical_power_consumed=0 W  mechanical_power_consumed_nominal_specify=off  mechanical_power_consumed_nominal_unit=W  mechanical_power_consumed_nominal_value=1  Tmeas=298.15 K  alpha=3.93e-3 1/K  alpha_cage=4.4e-3 1/K  stator_thermal_mass=100 J/K  rotor_thermal_mass=200 J/K  temperatureA_specify=off  temperatureA_priority=High  temperatureA=25 degC  temperatureA_nominal_specify=off  temperatureA_nominal_unit=degC  temperatureA_nominal_value=1  temperatureB_specify=off  temperatureB_priority=High  temperatureB=25 degC  temperatureB_nominal_specify=off  temperatureB_nominal_unit=degC  temperatureB_nominal_value=1  temperatureC_specify=off  temperatureC_priority=High  temperatureC=25 degC  temperatureC_nominal_specify=off  temperatureC_nominal_unit=degC  temperatureC_nominal_value=1  temperatureR_specify=off  temperatureR_priority=High  temperatureR=25 degC  temperatureR_nominal_specify=off  temperatureR_nominal_unit=degC  temperatureR_nominal_value=1
      settings: InternalSimscapePortConfiguration="{\"Bottom\":[],\"Left\":[{\"id\":\"R\",\"label\":\"R\",\"type\":\"foundation.mechanical.rotational.rotational\"},{\"id\":\"C\",\"label\":\"C\",\"type\":\"foundation.mechanical.rotational.rotational\"}],\"Right\":[{\"id\":\"pu_output\",\"label\":\"pu\",\"type\":\"output\"},{\"id\":\"N1\",\"label\":\"~1\",\"type\":\"foundation.electrical.three_phase\"},{\"id\":\"N2\",\"label\":\"~2\",\"type\":\"foundation.electrical.three_phase\"}],\"Top\":[]}"
  Electrical Reference1 : fl_lib/Electrical/Electrical Elements/Electrical Reference
  Generator : Scope  NumInputPorts=3
  Generator Sign Convention : Gain  Gain=-1
  Generator Sign Convention1 : Gain  Gain=-1
  Neutral Port (Three-Phase) : ee_lib/Connectors & References/Neutral Port (Three-Phase)  G_parasitic=1e-12 1/Ohm
      settings: InternalSimscapePortConfiguration="{\"Bottom\":[],\"Left\":[{\"id\":\"N\",\"label\":\"~\",\"type\":\"foundation.electrical.three_phase\"}],\"Right\":[{\"id\":\"n\",\"label\":\"n\",\"type\":\"foundation.electrical.electrical\"}],\"Top\":[]}"
  PS-Simulink Converter1 : nesl_utility/PS-Simulink Converter  PhysicalDomain=network_engine_domain  SubClassName=ps_output  LeftPortType=input  RightPortType=output  PseudoPeriodic=off  Frequencies=[]  VectorFormat=1-D array  Unit=1  AffineConversion=off
  PS-Simulink Converter2 : nesl_utility/PS-Simulink Converter  PhysicalDomain=network_engine_domain  SubClassName=ps_output  LeftPortType=input  RightPortType=output  PseudoPeriodic=off  Frequencies=[]  VectorFormat=1-D array  Unit=1  AffineConversion=off
  PS-Simulink Converter3 : nesl_utility/PS-Simulink Converter  PhysicalDomain=network_engine_domain  SubClassName=ps_output  LeftPortType=input  RightPortType=output  PseudoPeriodic=off  Frequencies=[]  VectorFormat=1-D array  Unit=1  AffineConversion=off
  Subsystem : Subsystem
  Conn2 : PMIOPort  Side=Right
  wires:
  PS-Simulink Converter3/1 -> Generator/3
  Generator Sign Convention1/1 -> Generator/2  "Reactive Power, pu"
  PS-Simulink Converter2/1 -> Generator Sign Convention/1
  Generator Sign Convention/1 -> Generator/1  "Real Power, pu"
  PS-Simulink Converter1/1 -> Generator Sign Convention1/1
  connections:
  ASM measurement1/RConn1 -- PS-Simulink Converter1/LConn1
  PS-Simulink Converter3/LConn1 -- ASM measurement2/RConn1
  Asynchronous Machine Squirrel Cage (fundamental)/RConn3 -- Neutral Port (Three-Phase)/LConn1
  Asynchronous Machine Squirrel Cage (fundamental)/RConn2 -- Conn2/RConn1
  ASM measurement/RConn1 -- PS-Simulink Converter2/LConn1
  Neutral Port (Three-Phase)/RConn1 -- Electrical Reference1/LConn1
  Subsystem/LConn1 -- Asynchronous Machine Squirrel Cage (fundamental)/LConn1
  Subsystem/LConn2 -- Asynchronous Machine Squirrel Cage (fundamental)/LConn2
  ASM measurement1/LConn1 -- ASM measurement2/LConn1 -- Asynchronous Machine Squirrel Cage (fundamental)/RConn1 -- ASM measurement/LConn1

== system IndustrialMicrogrid/MG1 Primary Substation/BESS and Controller ==
  CntrlRmIN : Inport
  PQref : Inport  Port=2
  Vref : Inport  Port=3
  f0 : Inport  Port=4
  BESS : Subsystem
      settings: PortSchema="{\"entries\":[{\"content\":{\"sides\":[{\"content\":{\"connectorIds\":[\"LConn1\"]},\"type\":\"ConnectorPlacement.EquallySpacedRectSide\",\"uuid\":\"67533fe0-854e-4cff-97db-4a2dd73ea00c\"},{\"content\":{\"connectorIds\":[\"In1\",\"In2\",\"In3\",\"In4\"],\"side\":\"RIGHT\"},\"type\":\"ConnectorPlacement.EquallySpacedRectSide\",\"uuid\":\"dbf34e3e-6cf0-48a4-951d-868729a6dadd\"},{\"content\":{\"side\":\"TOP\"},\"type\":\"ConnectorPlacement.EquallySpacedRectSide\",\"uuid\":\"e0bf98cd-b60e-4b50-bc9a-0e2d83d9ef47\"}]},\"type\":\"ConnectorPlacement.EquallySpacedConnector\",\"uuid\":\"edf752ef-de3e-4d7a-8ea9-04227b44108e\"}],\"packageUris\":[\"http://schema.mathworks.com/mf0/Connector/R2020b\"],\"version\":\"1.0\"}"
  "BESS Converter Measurement " : Subsystem
  BESS output filter and transformer : Subsystem
  ~ : PMIOPort  Side=Left
  mBESS : Outport
  wires:
  Vref/1 -> BESS/3(Vref)
  f0/1 -> BESS/4(f0)
  "BESS Converter Measurement "/1(mBESS) -> mBESS/1
  CntrlRmIN/1 -> BESS/1(CntrlRmIN1)
  PQref/1 -> BESS/2(PQref)
  connections:
  "BESS Converter Measurement "/LConn1 -- BESS output filter and transformer/RConn1
  "BESS Converter Measurement "/RConn1 -- ~/RConn1
  BESS output filter and transformer/LConn1 -- BESS/LConn1
